simulink model "simple_non_linear"  (R2019a)
settings: Solver=VariableStepAuto  StartTime=0.0  StopTime=10  RelTol=1e-3
settings Model: Creator=iyengar  LastModifiedBy=iyengar

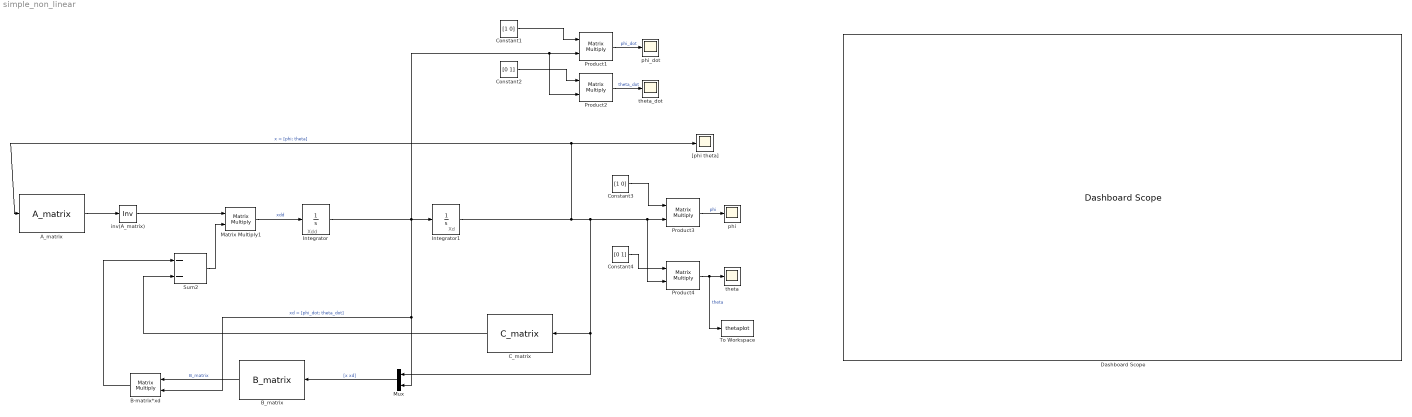
== system simple_non_linear ==
  note: Xdd
  note: Xd
  "A_matrix " : MATLABFcn  Description=matrix A. 2x2  MATLABFcn=A_matrix  OutputDimensions=[2, 2]  Output1D=off
  B-matrix*xd : Product  Multiplication=Matrix(*)
  B_matrix : MATLABFcn  MATLABFcn=B_matrix  Output1D=off
  C_matrix : MATLABFcn  MATLABFcn=C_matrix  Output1D=off
  Constant1 : Constant  Value=[1 0]  VectorParams1D=off
  Constant2 : Constant  Value=[0 1]  VectorParams1D=off
  Constant3 : Constant  Value=[1 0]  VectorParams1D=off
  Constant4 : Constant  Value=[0 1]  VectorParams1D=off
  Dashboard Scope : DashboardScope
  Integrator : Integrator  InitialCondition=[0; 0]
  Integrator1 : Integrator  InitialCondition=[0; 0.5]
  Matrix Multiply1 : Product  Multiplication=Matrix(*)
  Mux : Mux  Inputs=2
  Product{1..4} (4 alike) : Product  Multiplication=Matrix(*)
  Sum2 : Sum  Inputs=--
  To Workspace : ToWorkspace  VariableName=thetaplot  SaveFormat=Timeseries  SampleTime=-1
  "[phi theta]" : Scope
  inv(A_matrix) : Product  Inputs=/  Multiplication=Matrix(*)
  phi : Scope
  phi_dot : Scope
  theta : Scope
  theta_dot : Scope
  wires:
  C_matrix/1 -> Sum2/2
  B-matrix*xd/1 -> Sum2/1
  Product3/1 -> phi/1  "phi"
  Constant4/1 -> Product4/1
  Product4/1 -> To Workspace/1, theta/1  "theta"
  Integrator1/1 -> "A_matrix "/1, "[phi theta]"/1, Mux/1, C_matrix/1, Product4/2, Product3/2  "x = [phi; theta]"
  B_matrix/1 -> B-matrix*xd/1  "B_matrix"
  inv(A_matrix)/1 -> Matrix Multiply1/1
  Constant2/1 -> Product2/1
  "A_matrix "/1 -> inv(A_matrix)/1
  Sum2/1 -> Matrix Multiply1/2
  Mux/1 -> B_matrix/1  "[x xd]"
  Product2/1 -> theta_dot/1  "theta_dot"
  Constant3/1 -> Product3/1
  Integrator/1 -> Product2/2, Product1/2, Integrator1/1, Mux/2, B-matrix*xd/2  "xd = [phi_dot; theta_dot]"
  Constant1/1 -> Product1/1
  Matrix Multiply1/1 -> Integrator/1  "xdd"
  Product1/1 -> phi_dot/1  "phi_dot"
